simulink model "LineAnalyser"  (R2015b)
settings: configuration reference "ControlConfig" (kept outside this file)
InitFcn:
  | ControlInit;
StopFcn:
  | LinePlot;
undefined symbols (not defined in the file or in its folder): Fnom, magnitude, Rad2Deg, Ts
libraries: powerlib x13, simulink x1, powerlib_meascontrol x1
settings Model: Creator=Emilio  LastModifiedBy=Emilio
settings ConfigSetRef: SourceLocation=Base Workspace

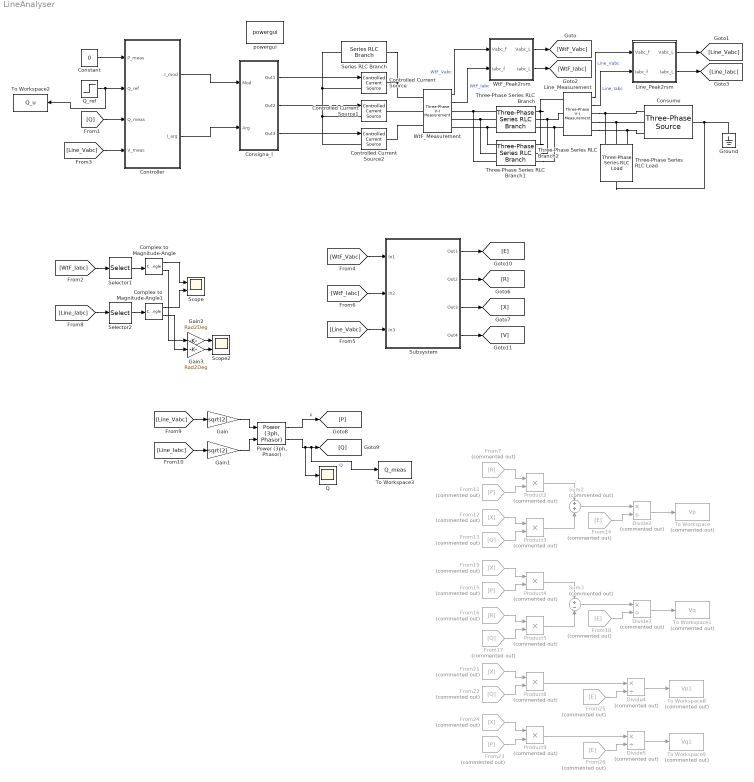
== system LineAnalyser ==
  Complex to Magnitude-Angle : ComplexToMagnitudeAngle
  Complex to Magnitude-Angle1 : ComplexToMagnitudeAngle
  Consigna_I : Subsystem
  Constant : Constant  Value=0
  Consume : powerlib/Electrical Sources/Three-Phase Source  InternalConnection=Yn  VoltagePhases=off  Voltage=220e3  PhaseAngle=0  Voltage_phases=[25e3 25e3 25e3]/sqrt(3)  PhaseAngles_phases=[0 -120 +120]  Frequency=Fnom  NonIdealSource=on  SpecifyImpedance=on  Resistance=0.8929  Inductance=16.58e-3  ShortCircuitLevel=100e6  BaseVoltage=25e3  XRratio=7  BusType=swing  Pref=10e3  Qref=0  Prefabc=[10e3, 10e3, 10e3]  Qrefabc=[0, 0, 0]  Qmin=-inf  Qmax=inf
  Controlled Current Source : powerlib/Electrical Sources/Controlled Current Source  Initialize=on  Source_Type=AC  Amplitude=1  Phase=1  Frequency=Fnom  Measurements=None
  Controlled Current Source1 : powerlib/Electrical Sources/Controlled Current Source  Initialize=on  Source_Type=AC  Amplitude=1  Phase=1  Frequency=Fnom  Measurements=None
  Controlled Current Source2 : powerlib/Electrical Sources/Controlled Current Source  Initialize=on  Source_Type=AC  Amplitude=1  Phase=1  Frequency=Fnom  Measurements=None
  Controller : Subsystem
  Divide{2..5} (4 alike) : Product  Commented=on  Inputs=*/
  From11 : From  Commented=on  GotoTag=P
  From{12,19,21,24} (4 alike) : From  Commented=on  GotoTag=X
  From13 : From  Commented=on  GotoTag=Q
  From{14,18,25..26} (4 alike) : From  Commented=on  GotoTag=E
  From15 : From  Commented=on  GotoTag=P
  From16 : From  Commented=on  GotoTag=R
  From17 : From  Commented=on  GotoTag=Q
  From22 : From  Commented=on  GotoTag=Q
  From23 : From  Commented=on  GotoTag=P
  From7 : From  Commented=on  GotoTag=R
  Gain : Gain  Gain=sqrt(2)
  Gain1 : Gain  Gain=sqrt(2)
  Gain2 : Gain  Gain=Rad2Deg
  Gain3 : Gain  Gain=Rad2Deg
  Ground : powerlib/Elements/Ground  LConnTagsString=a
  Line_Measurement : powerlib/Measurements/Three-Phase V-I Measurement  VoltageMeasurement=phase-to-ground  SetLabelV=off  LabelV=WtF_Vabc  Vpu=off  VpuLL=off  CurrentMeasurement=yes  SetLabelI=off  LabelI=WtF_Iabc  Ipu=off  Pbase=100e6  Vbase=500e3  OutputType=Complex  PhasorSimulation=on  PSBequivalent=0
  Line_Peak2rsm : Subsystem
  "Power (3ph, Phasor)" : powerlib_meascontrol/Measurements/Power (3ph, Phasor)
  Product{2..5,8..9} (6 alike) : Product  Commented=on
  Q : Scope
  Q_ref : Step  Time=0.02  After=4e6  SampleTime=0
  Scope : Scope  NumInputPorts=2
  Scope2 : Scope  NumInputPorts=2
  Selector1 : Selector  InputPortWidth=3  IndexOptions=Index vector (dialog)  Indices=[1]  OutputSizes=1
  Selector2 : Selector  InputPortWidth=3  IndexOptions=Index vector (dialog)  Indices=[3]  OutputSizes=1
  Series RLC Branch : powerlib/Elements/Series RLC Branch  LConnTagsString=__new0  RConnTagsString=__new0  BranchType=R  Resistance=10e12  Inductance=1e-3  SetiL0=off  InitialCurrent=0  Capacitance=1e-6  Setx0=off  InitialVoltage=0  Measurements=None
  Subsystem : Subsystem
  Sum2 : Sum  Commented=on  Inputs=+|+
  Sum3 : Sum  Commented=on  Inputs=+|-
  Three-Phase Series RLC Branch : powerlib/Elements/Three-Phase Series RLC Branch  LConnTagsString=A|B|C  RConnTagsString=A|B|C  BranchType=RL  Resistance=10  Inductance=0  Capacitance=0  Measurements=None
  Three-Phase Series RLC Branch1 : powerlib/Elements/Three-Phase Series RLC Branch  LConnTagsString=A|B|C  RConnTagsString=A|B|C  BranchType=R  Resistance=10  Inductance=0  Capacitance=0  Measurements=Branch currents
  Three-Phase Series RLC Branch2 : powerlib/Elements/Three-Phase Series RLC Branch  LConnTagsString=A|B|C  RConnTagsString=A|B|C  BranchType=R  Resistance=10  Inductance=0  Capacitance=0  Measurements=None
  Three-Phase Series RLC Load : powerlib/Elements/Three-Phase Series RLC Load  LConnTagsString=A|B|C  RConnTagsString=N  Configuration=Y (neutral)  NominalVoltage=1000  Vabc=[1e3 1e3 1e3]  Vabcp=[1e3 1e3 1e3]  NominalFrequency=Fnom  UnbalancedPower=off  ActivePower=0.1  InductivePower=0  CapacitivePower=0  Pabc=[10e3 9e3 11e3]  QLabc=[100 90 110]  QCabc=[100 90 110]  Pabcp=[10e3 9e3 11e3]  QLabcp=[100 90 110]  QCabcp=[100 90 110]  Measurements=None  LoadType=constant Z
  To Workspace : ToWorkspace  Commented=on  VariableName=Vp  SampleTime=-1
  To Workspace1 : ToWorkspace  Commented=on  VariableName=Vq  SampleTime=-1
  To Workspace2 : ToWorkspace  VariableName=Q_u  SampleTime=Ts
  To Workspace3 : ToWorkspace  VariableName=Q_meas  SaveFormat=Structure With Time  SampleTime=-1
  To Workspace8 : ToWorkspace  Commented=on  VariableName=Vp1  SampleTime=-1
  To Workspace9 : ToWorkspace  Commented=on  VariableName=Vq1  SampleTime=-1
  WtF_Measurement : powerlib/Measurements/Three-Phase V-I Measurement  VoltageMeasurement=phase-to-ground  SetLabelV=off  LabelV=WtF_Vabc  Vpu=off  VpuLL=off  CurrentMeasurement=yes  SetLabelI=off  LabelI=WtF_Iabc  Ipu=off  Pbase=100e6  Vbase=500e3  OutputType=Complex  PhasorSimulation=on  PSBequivalent=0
  WtF_Peak2rsm : Subsystem
  powergui : powerlib/powergui  Priority=1  SimulationMode=Phasor  SolverType=Backward Euler  SampleTime=50e-6  frequency=Fnom  SPID=off  DisableSnubberDevices=off  DisableRonSwitches=off  DisableVfSwitches=off  SwTol=0  DisplayEquations=off  Interpol=off  ExternalGateDelay=off  methode=off  Ts=10  FunctionMessages=off  echomessages=off  HookPort=off  EnableUseOfTLC=off  x0status=blocks  frequencyindice=50  Pbase=100e6  ErrMax=1e-4  Iterations=50  UnitsV=kV  UnitsW=MW  buscounter=0  RestoreLinks=warning  ResistiveCurrentMeasurement=off  Frange=[0:2:500]  Ylog=off  Xlog=on  ShowGrid=off  save=off  variable=ZData  structure=0  ZoomFFT=off  StartTime=0.0  cycles=1  DisplayStyle=1  fundamental=60  FreqAxis=off  MaxFrequency=1000  frequencyindicesteady=1  RmsSteady=1  display=off
  wires:
  Consigna_I/1(Out1) -> Controlled Current Source/1
  Consigna_I/2(Out2) -> Controlled Current Source1/1
  Consigna_I/3(Out3) -> Controlled Current Source2/1
  [Line_Vabc] -> Gain/1
  [Line_Iabc] -> Gain1/1
  "Power (3ph, Phasor)"/1 -> [P]  "P"
  "Power (3ph, Phasor)"/2 -> Q/1, To Workspace3/1, [Q]  "Q"
  From7/1 -> Product2/1
  From11/1 -> Product2/2
  From12/1 -> Product3/1
  From13/1 -> Product3/2
  Product2/1 -> Sum2/1
  Product3/1 -> Sum2/2
  Sum2/1 -> Divide2/1
  From14/1 -> Divide2/2
  From19/1 -> Product4/1
  From15/1 -> Product4/2
  From16/1 -> Product5/1
  From17/1 -> Product5/2
  Product4/1 -> Sum3/1
  Product5/1 -> Sum3/2
  Sum3/1 -> Divide3/1
  From18/1 -> Divide3/2
  Divide3/1 -> To Workspace1/1
  Divide2/1 -> To Workspace/1
  From21/1 -> Product8/1
  From22/1 -> Product8/2
  From24/1 -> Product9/1
  From23/1 -> Product9/2
  Product8/1 -> Divide4/1
  From25/1 -> Divide4/2
  Product9/1 -> Divide5/1
  From26/1 -> Divide5/2
  Divide5/1 -> To Workspace9/1
  [WtF_Vabc] -> Subsystem/1(In1)
  [WtF_Iabc] -> Subsystem/2(In2)
  [Line_Vabc] -> Subsystem/3(In3)
  Subsystem/1(Out1) -> [E]
  Subsystem/2(Out2) -> [R]
  Subsystem/3(Out3) -> [X]
  Subsystem/4(Out4) -> [V]
  Line_Measurement/1 -> Line_Peak2rsm/1(Vabc_f)  "Line_Vabc"
  Line_Measurement/2 -> Line_Peak2rsm/2(Iabc_f)  "Line_Iabc"
  Line_Peak2rsm/1(Vabc_L) -> [Line_Vabc]
  Line_Peak2rsm/2(Iabc_L) -> [Line_Iabc]
  WtF_Peak2rsm/1(Vabc_L) -> [WtF_Vabc]
  WtF_Peak2rsm/2(Iabc_L) -> [WtF_Iabc]
  WtF_Measurement/1 -> WtF_Peak2rsm/1(Vabc_f)  "WtF_Vabc"
  WtF_Measurement/2 -> WtF_Peak2rsm/2(Iabc_f)  "WtF_Iabc"
  Divide4/1 -> To Workspace8/1
  Gain/1 -> "Power (3ph, Phasor)"/1
  Gain1/1 -> "Power (3ph, Phasor)"/2
  [Q] -> Controller/3(Q_meas)
  Constant/1 -> Controller/1(P_meas)
  [Line_Vabc] -> Controller/4(V_meas)
  Q_ref/1 -> To Workspace2/1, Controller/2(Q_ref)
  Controller/2(I_arg) -> Consigna_I/2(Arg)
  Controller/1(I_mod) -> Consigna_I/1(Mod)
  [WtF_Iabc] -> Selector1/1
  [Line_Iabc] -> Selector2/1
  Complex to Magnitude-Angle/1 -> Scope/1
  Complex to Magnitude-Angle1/1 -> Scope/2
  Selector2/1 -> Complex to Magnitude-Angle1/1
  Selector1/1 -> Complex to Magnitude-Angle/1
  Gain2/1 -> Scope2/1
  Gain3/1 -> Scope2/2
  Complex to Magnitude-Angle1/2 -> Gain3/1
  Complex to Magnitude-Angle/2 -> Gain2/1
  connections:
  WtF_Measurement/LConn3 -- Controlled Current Source2/RConn1
  WtF_Measurement/LConn2 -- Controlled Current Source1/RConn1
  Controlled Current Source2/LConn1 -- Series RLC Branch/LConn1 -- Controlled Current Source/LConn1 -- Controlled Current Source1/LConn1
  Line_Measurement/LConn3 -- Three-Phase Series RLC Branch1/RConn3 -- Three-Phase Series RLC Branch/RConn3
  Three-Phase Series RLC Branch/RConn2 -- Three-Phase Series RLC Branch1/RConn2 -- Line_Measurement/LConn2
  Three-Phase Series RLC Branch/RConn1 -- Three-Phase Series RLC Branch1/RConn1 -- Line_Measurement/LConn1
  Line_Measurement/RConn1 -- Three-Phase Series RLC Load/LConn1 -- Consume/RConn3
  Line_Measurement/RConn2 -- Three-Phase Series RLC Load/LConn2 -- Consume/RConn2
  Three-Phase Series RLC Load/RConn1 -- Consume/LConn1 -- Ground/LConn1
  Three-Phase Series RLC Branch/LConn2 -- WtF_Measurement/RConn2 -- Three-Phase Series RLC Branch1/LConn2
  Three-Phase Series RLC Branch/LConn1 -- WtF_Measurement/RConn1 -- Three-Phase Series RLC Branch1/LConn3
  Three-Phase Series RLC Branch/LConn3 -- Three-Phase Series RLC Branch1/LConn1 -- WtF_Measurement/RConn3
  Line_Measurement/RConn3 -- Three-Phase Series RLC Load/LConn3 -- Consume/RConn1
  Series RLC Branch/RConn1 -- WtF_Measurement/LConn1 -- Controlled Current Source/RConn1

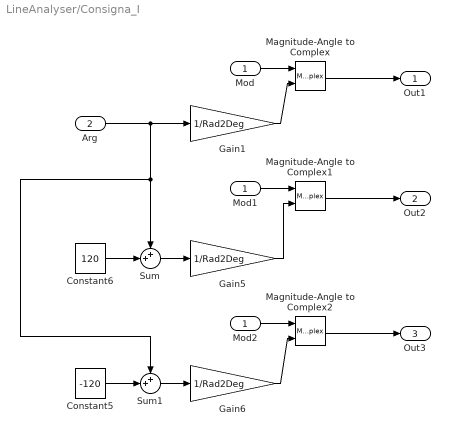
== system LineAnalyser/Consigna_I ==
  Mod : Inport
  Arg : Inport  Port=2
  Constant5 : Constant  Value=-120
  Constant6 : Constant  Value=120
  Gain1 : Gain  Gain=1/Rad2Deg
  Gain5 : Gain  Gain=1/Rad2Deg
  Gain6 : Gain  Gain=1/Rad2Deg
  Magnitude-Angle to Complex : MagnitudeAngleToComplex
  Magnitude-Angle to Complex1 : MagnitudeAngleToComplex
  Magnitude-Angle to Complex2 : MagnitudeAngleToComplex
  Mod1 : InportShadow
  Mod2 : InportShadow
  Sum : Sum  Inputs=++|
  Sum1 : Sum  Inputs=++|
  Out1 : Outport
  Out2 : Outport  Port=2
  Out3 : Outport  Port=3
  wires:
  Magnitude-Angle to Complex/1 -> Out1/1
  Magnitude-Angle to Complex1/1 -> Out2/1
  Magnitude-Angle to Complex2/1 -> Out3/1
  Gain5/1 -> Magnitude-Angle to Complex1/2
  Gain6/1 -> Magnitude-Angle to Complex2/2
  Mod2/1 -> Magnitude-Angle to Complex2/1
  Mod1/1 -> Magnitude-Angle to Complex1/1
  Mod/1 -> Magnitude-Angle to Complex/1
  Arg/1 -> Gain1/1, Sum/1, Sum1/1
  Sum1/1 -> Gain6/1
  Constant5/1 -> Sum1/2
  Sum/1 -> Gain5/1
  Constant6/1 -> Sum/2
  Gain1/1 -> Magnitude-Angle to Complex/2

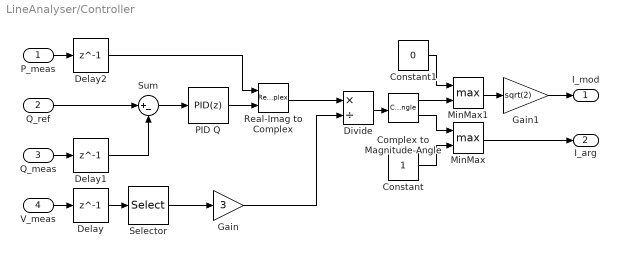
== system LineAnalyser/Controller ==
  P_meas : Inport
  Q_ref : Inport  Port=2
  Q_meas : Inport  Port=3
  V_meas : Inport  Port=4
      settings: SignalType=complex
  Complex to Magnitude-Angle : ComplexToMagnitudeAngle
  Constant : Constant
  Constant1 : Constant  Value=0
  Delay : Delay  DelayLength=1
  Delay1 : Delay  DelayLength=1
  Delay2 : Delay  DelayLength=1
  Divide : Product  Inputs=*/
  Gain : Gain  Gain=3
  Gain1 : Gain  Gain=sqrt(2)
  MinMax : MinMax  Function=max  Inputs=2
  MinMax1 : MinMax  Function=max  Inputs=2
  PID Q : simulink/Continuous/PID Controller  Controller=PID  TimeDomain=Discrete-time  SampleTime=Ts  IntegratorMethod=Forward Euler  FilterMethod=Forward Euler  Form=Parallel  UseFilter=on  ControllerParametersSource=internal  P=0.2  I=0.9  D=0  N=100  InitialConditionSource=internal  InitialConditionForIntegrator=0  InitialConditionForFilter=0  ExternalReset=none  LimitOutput=off  UpperSaturationLimit=inf  LowerSaturationLimit=-inf  LinearizeAsGain=off  AntiWindupMode=none  Kb=1  TrackingMode=off  Kt=1  PParamMin=[]  PParamMax=[]  IParamMin=[]  IParamMax=[]  DParamMin=[]  DParamMax=[]  NParamMin=[]  NParamMax=[]  KbParamMin=[]  KbParamMax=[]  KtParamMin=[]  KtParamMax=[]  POutMin=[]  POutMax=[]  IOutMin=[]  IOutMax=[]  DOutMin=[]  DOutMax=[]  NOutMin=[]  NOutMax=[]  KbOutMin=[]  KbOutMax=[]  KtOutMin=[]  KtOutMax=[]  IntegratorOutMin=[]  IntegratorOutMax=[]  FilterOutMin=[]  FilterOutMax=[]  SumOutMin=[]  SumOutMax=[]  SumI1OutMin=[]  SumI1OutMax=[]  SumI2OutMin=[]  SumI2OutMax=[]  SumI3OutMin=[]  SumI3OutMax=[]  SumDOutMin=[]  SumDOutMax=[]  SaturationOutMin=[]  SaturationOutMax=[]  IntegratorContinuousStateAttributes=''  IntegratorStateMustResolveToSignalObject=off  IntegratorRTWStateStorageClass=Auto  FilterContinuousStateAttributes=''  FilterStateMustResolveToSignalObject=off  FilterRTWStateStorageClass=Auto  DifferentiatorICPrevScaledInput=0  DifferentiatorOutMin=[]  DifferentiatorOutMax=[]
  Real-Imag to Complex : RealImagToComplex
  Selector : Selector  InputPortWidth=3  IndexOptions=Index vector (dialog)  Indices=[1 ]  OutputSizes=1
  Sum : Sum  Inputs=|+-
  I_mod : Outport
  I_arg : Outport  Port=2
  wires:
  Q_ref/1 -> Sum/1
  Sum/1 -> PID Q/1
  Q_meas/1 -> Delay1/1
  PID Q/1 -> Real-Imag to Complex/2
  P_meas/1 -> Delay2/1
  V_meas/1 -> Delay/1
  Divide/1 -> Complex to Magnitude-Angle/1
  Selector/1 -> Gain/1
  Gain/1 -> Divide/2
  Constant/1 -> MinMax/2
  Complex to Magnitude-Angle/2 -> MinMax/1
  Delay/1 -> Selector/1
  Delay1/1 -> Sum/2
  Delay2/1 -> Real-Imag to Complex/1
  Complex to Magnitude-Angle/1 -> MinMax1/2
  MinMax1/1 -> Gain1/1
  Constant1/1 -> MinMax1/1
  Gain1/1 -> I_mod/1
  Real-Imag to Complex/1 -> Divide/1
  MinMax/1 -> I_arg/1

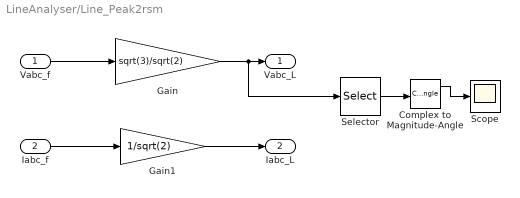
== system LineAnalyser/Line_Peak2rsm ==
  Vabc_f : Inport
  Iabc_f : Inport  Port=2
  Complex to Magnitude-Angle : ComplexToMagnitudeAngle
  Gain : Gain  Gain=sqrt(3)/sqrt(2)
  Gain1 : Gain  Gain=1/sqrt(2)
  Scope : Scope
  Selector : Selector  InputPortWidth=3  IndexOptions=Index vector (dialog)  Indices=[1]  OutputSizes=1
  Vabc_L : Outport
  Iabc_L : Outport  Port=2
  wires:
  Gain1/1 -> Iabc_L/1
  Gain/1 -> Selector/1, Vabc_L/1
  Vabc_f/1 -> Gain/1
  Iabc_f/1 -> Gain1/1
  Complex to Magnitude-Angle/1 -> Scope/1
  Selector/1 -> Complex to Magnitude-Angle/1

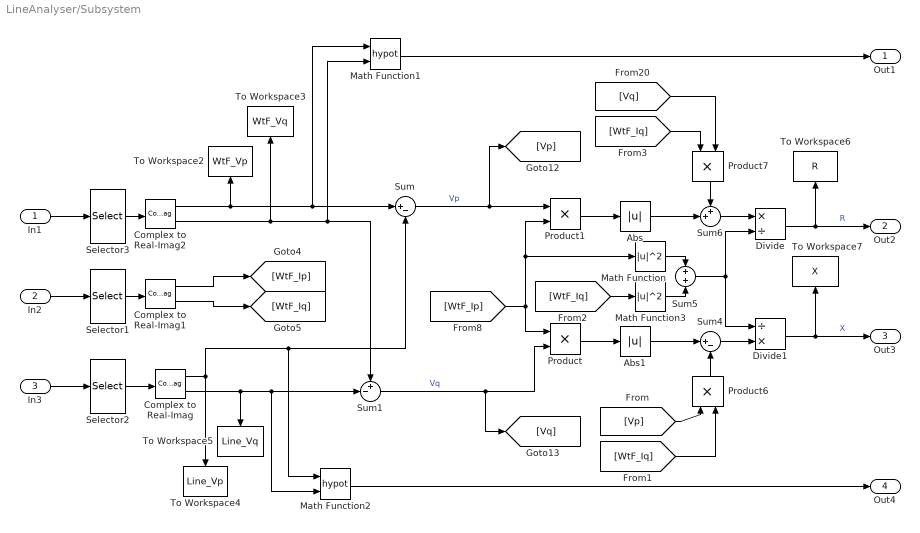
== system LineAnalyser/Subsystem ==
  In1 : Inport
  In2 : Inport  Port=2
  In3 : Inport  Port=3
  Abs : Abs
  Abs1 : Abs
  Complex to Real-Imag : ComplexToRealImag
  Complex to Real-Imag1 : ComplexToRealImag
  Complex to Real-Imag2 : ComplexToRealImag
  Divide : Product  Inputs=*/
  Divide1 : Product  Inputs=/*
  Math Function : Math  Operator=magnitude^2  SaturateOnIntegerOverflow=on
  Math Function1 : Math  Operator=hypot  SaturateOnIntegerOverflow=on
  Math Function2 : Math  Operator=hypot  SaturateOnIntegerOverflow=on
  Math Function3 : Math  Operator=magnitude^2  SaturateOnIntegerOverflow=on
  Product{,1,6..7} (4 alike) : Product
  Selector1 : Selector  InputPortWidth=3  IndexOptions=Index vector (dialog)  Indices=[1 ]  OutputSizes=1
  Selector2 : Selector  InputPortWidth=3  IndexOptions=Index vector (dialog)  Indices=[1 ]  OutputSizes=1
  Selector3 : Selector  InputPortWidth=3  IndexOptions=Index vector (dialog)  Indices=[1 ]  OutputSizes=1
  Sum : Sum  Inputs=|+-
  Sum1 : Sum  Inputs=+-|
  Sum4 : Sum  Inputs=|+-
  Sum5 : Sum  Inputs=+|+
  Sum6 : Sum  Inputs=++|
  To Workspace2 : ToWorkspace  VariableName=WtF_Vp  SampleTime=-1
  To Workspace3 : ToWorkspace  VariableName=WtF_Vq  SampleTime=-1
  To Workspace4 : ToWorkspace  VariableName=Line_Vp  SampleTime=-1
  To Workspace5 : ToWorkspace  VariableName=Line_Vq  SampleTime=-1
  To Workspace6 : ToWorkspace  VariableName=R  SampleTime=-1
  To Workspace7 : ToWorkspace  VariableName=X  SampleTime=-1
  Out1 : Outport
  Out2 : Outport  Port=2
  Out3 : Outport  Port=3
  Out4 : Outport  Port=4
  wires:
  In2/1 -> Selector1/1
  In3/1 -> Selector2/1
  In1/1 -> Selector3/1
  Complex to Real-Imag2/2 -> Sum1/1, Math Function1/2, To Workspace3/1
  Complex to Real-Imag1/1 -> [WtF_Ip]
  Complex to Real-Imag/1 -> Math Function2/1, Sum/2, To Workspace4/1
  Math Function1/1 -> Out1/1
  Math Function2/1 -> Out4/1
  Complex to Real-Imag/2 -> Math Function2/2, Sum1/2, To Workspace5/1
  [WtF_Ip] -> Product1/2, Math Function/1, Product/1
  Complex to Real-Imag1/2 -> [WtF_Iq]
  Complex to Real-Imag2/1 -> Math Function1/1, Sum/1, To Workspace2/1
  Divide/1 -> Out2/1, To Workspace6/1  "R"
  Sum1/1 -> [Vq], Product/2  "Vq"
  Divide1/1 -> Out3/1, To Workspace7/1  "X"
  Product/1 -> Abs1/1
  [Vq] -> Product7/2
  [WtF_Iq] -> Math Function3/1
  Sum5/1 -> Divide/2, Divide1/1
  Math Function/1 -> Sum5/1
  Selector2/1 -> Complex to Real-Imag/1
  [WtF_Iq] -> Product6/2
  Math Function3/1 -> Sum5/2
  Sum4/1 -> Divide1/2
  Sum6/1 -> Divide/1
  Sum/1 -> [Vp], Product1/1  "Vp"
  [WtF_Iq] -> Product7/1
  Product6/1 -> Sum4/2
  [Vp] -> Product6/1
  Product1/1 -> Abs/1
  Product7/1 -> Sum6/1
  Abs1/1 -> Sum4/1
  Abs/1 -> Sum6/2
  Selector1/1 -> Complex to Real-Imag1/1
  Selector3/1 -> Complex to Real-Imag2/1

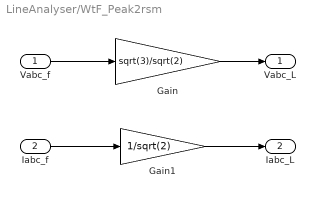
== system LineAnalyser/WtF_Peak2rsm ==
  Vabc_f : Inport
  Iabc_f : Inport  Port=2
  Gain : Gain  Gain=sqrt(3)/sqrt(2)
  Gain1 : Gain  Gain=1/sqrt(2)
  Vabc_L : Outport
  Iabc_L : Outport  Port=2
  wires:
  Iabc_f/1 -> Gain1/1
  Vabc_f/1 -> Gain/1
  Gain/1 -> Vabc_L/1
  Gain1/1 -> Iabc_L/1
